simulink model "sim_test_outputFB"  (R2016a)
settings: Solver=ode3  StartTime=0.0  StopTime=Tsim  FixedStep=Ts  RelTol=1e-3
undefined symbols (not defined in the file): dist, Ksys, P2, ref, Tdist, Tref, x0, xK0
settings Model: Creator=Matti  LastModifiedBy=Matti

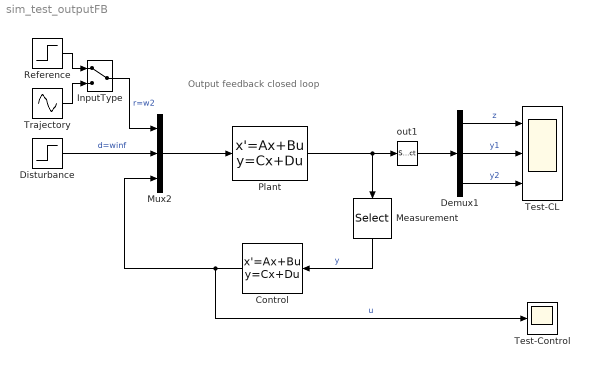
== system sim_test_outputFB ==
  note: Output feedback closed loop
  Control : StateSpace  A=Ksys.A  B=Ksys.B  C=Ksys.C  D=Ksys.D  X0=xK0
  Demux1 : Demux  Outputs=3
  Disturbance : Step  Time=Tdist  After=dist  SampleTime=0
  InputType : ManualSwitch
  Measurement : Selector  InputPortWidth=4  IndexOptions=Index vector (dialog)  Indices=[3 4]  OutputSizes=1
  Mux2 : Mux  Inputs=3
  Plant : StateSpace  A=P2.A  B=P2.B  C=P2.C  D=P2.D  X0=x0
  Reference : Step  Time=Tref  After=ref  SampleTime=0
  Test-CL : Scope  NumInputPorts=3
  Test-Control : Scope
  Trajectory : Sin  Frequency=0.5  SampleTime=0
  out1 : Selector  InputPortWidth=4  IndexOptions=Index vector (dialog)  Indices=[1 3 4]  OutputSizes=1
  wires:
  Disturbance/1 -> Mux2/2  "d=winf"
  Measurement/1 -> Control/1  "y"
  Plant/1 -> Measurement/1, out1/1
  Control/1 -> Test-Control/1, Mux2/3  "u"
  Demux1/3 -> Test-CL/3  "y2"
  Demux1/2 -> Test-CL/2  "y1"
  Mux2/1 -> Plant/1
  Reference/1 -> InputType/1
  InputType/1 -> Mux2/1  "r=w2"
  Trajectory/1 -> InputType/2
  Demux1/1 -> Test-CL/1  "z"
  out1/1 -> Demux1/1
